simulink model "Solar_Panel"  (R2025b)
settings: Solver=VariableStepAuto  StartTime=0.0  StopTime=3600  RelTol=1e-3
undefined symbols (not defined in the file): J, Kd, Kf, Kg, Kt, L, R, sunPosition
libraries: slpidlib x1
settings Model: Creator=night  LastModifiedBy=night
settings DataIOCC: ExternalInput=[sunTime, sunPosition]  LoadExternalInput=on

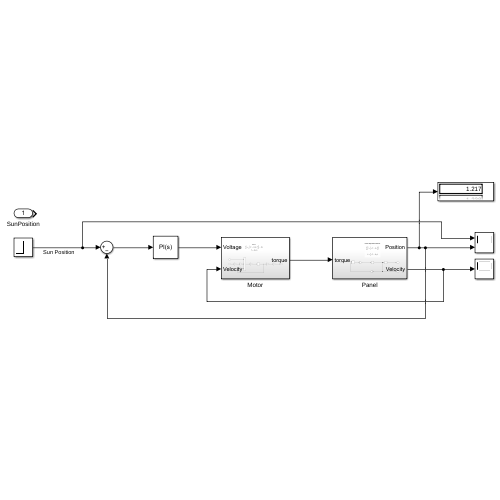
[thumbnail: Simulink's stored preview of the top-level diagram]
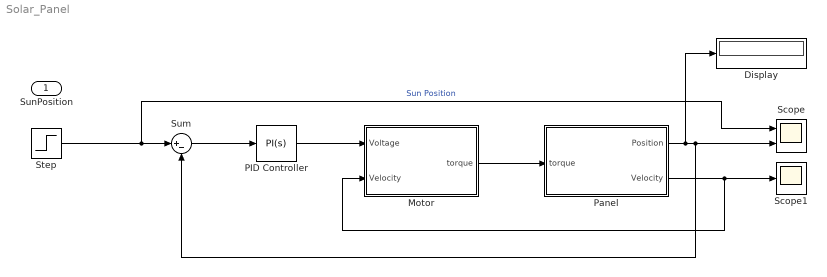
== system Solar_Panel ==
  SunPosition : Inport
  Display : Display
  Motor : Subsystem
  PID Controller : slpidlib/PID Controller  Controller=PI  Form=Parallel  TimeDomain=Continuous-time  UseExternalTs=off  SampleTime=-1  IntegratorMethod=Forward Euler  FilterMethod=Forward Euler  ControllerParametersSource=internal  P=240  I=180  UseKiTs=off  D=0  UseExternalDerivativeSource=off  N=100  UseFilter=on  TunerSelectOption=Transfer Function Based (PID Tuner App)  InitialConditionSource=internal  InitialConditionForIntegrator=0  InitialConditionForFilter=0  DifferentiatorICPrevScaledInput=0  ExternalReset=none  TrackingMode=off  Kt=1  LimitOutput=off  SatLimitsSource=internal  UpperSaturationLimit=inf  LowerSaturationLimit=-inf  LinearizeAsGain=on  AntiWindupMode=none  Kb=1  LimitIntegrator=off  UpperIntegratorSaturationLimit=inf  LowerIntegratorSaturationLimit=-inf  POutMin=[]  POutMax=[]  IOutMin=[]  IOutMax=[]  DOutMin=[]  DOutMax=[]  NOutMin=[]  NOutMax=[]  SumOutMin=[]  SumOutMax=[]  SaturationOutMin=[]  SaturationOutMax=[]  PParamMin=[]  PParamMax=[]  IParamMin=[]  IParamMax=[]  DParamMin=[]  DParamMax=[]  NParamMin=[]  NParamMax=[]  KbParamMin=[]  KbParamMax=[]  KtParamMin=[]  KtParamMax=[]  KbOutMin=[]  KbOutMax=[]  KtOutMin=[]  KtOutMax=[]  IntegratorOutMin=[]  IntegratorOutMax=[]  FilterOutMin=[]  FilterOutMax=[]  SumI1OutMin=[]  SumI1OutMax=[]  SumI2OutMin=[]  SumI2OutMax=[]  SumI3OutMin=[]  SumI3OutMax=[]  SumI4OutMin=[]  SumI4OutMax=[]  SumDOutMin=[]  SumDOutMax=[]  DifferentiatorOutMin=[]  DifferentiatorOutMax=[]  FilterDiffOutCoefMin=[]  FilterDiffOutCoefMax=[]  ReciprocalOutMin=[]  ReciprocalOutMax=[]  SumDenOutMin=[]  SumDenOutMax=[]  SumNumOutMin=[]  SumNumOutMax=[]  DivideOutMin=[]  DivideOutMax=[]  UdiffTsProdOutMin=[]  UdiffTsProdOutMax=[]  NTsProdOutMin=[]  NTsProdOutMax=[]  UintegralTsProdOutMin=[]  UintegralTsProdOutMax=[]  UngainTsProdOutMin=[]  UngainTsProdOutMax=[]  ClampingZeroOutDataTypeStr=Inherit: Inherit via back propagation  ClampingZeroOutMin=[]  ClampingZeroOutMax=[]  FilterDenConstantOutDataTypeStr=Inherit: Inherit via back propagation  FilterDenConstantOutMin=[]  FilterDenConstantOutMax=[]  PCopyOutDataTypeStr=Inherit: Inherit via back propagation  PCopyOutMin=[]  PCopyOutMax=[]  NCopyOutDataTypeStr=Inherit: Inherit via back propagation  NCopyOutMin=[]  NCopyOutMax=[]  IntegratorContinuousStateAttributes=''  IntegratorStateMustResolveToSignalObject=off  IntegratorRTWStateStorageClass=Auto  FilterContinuousStateAttributes=''  FilterStateMustResolveToSignalObject=off  FilterRTWStateStorageClass=Auto  ParallelPVariant=InternalParameters  IdealPVariant=Disabled  IVariant=InternalParameters  DVariant=Disabled  IntegratorVariant=Continuous  SatVariant=Disabled  AWVariant=Passthrough  PCopyVariant=Disabled  TRVariant=Disabled  FdbkBlocksVariant=Forward  IdealPFdbkVariant=Disabled  SatFdbkVariant=Disabled  DerivativeFilterVariant=Disabled  NVariant=Disabled  NCopyVariant=Disabled_SignalSpec  FilterICVariant=Disabled  IntegratorICVariant=InternalICs  ExternalResetVariant=Disabled  TRSumVariant=Passthrough  SumFdbkVariant=Disabled  SumVariant=Sum_PI  TsampFilterVariant=InternalTs  TsampNgainVariant=Passthrough  TsampIntegralVariant=Disabled_SignalSpec  ExternalSaturationOutDataTypeStr=Inherit: Same as second input  DerivativeSourceVariant=Disabled  PreIntVariant=InternalPreInt
  Panel : Subsystem
  Scope : Scope  NumInputPorts=2
      settings: Title=Solar Panel's Motor and Panel Assembly  ActiveDisplayYMinimum=-1  ActiveDisplayYMaximum=1
  Scope1 : Scope
      settings: ActiveDisplayYMinimum=-1  ActiveDisplayYMaximum=1
  Step : Step  After=sunPosition  SampleTime=0
  Sum : Sum  Inputs=|+-
  wires:
  Motor/1(torque) -> Panel/1(torque)
  Panel/1(Position) -> Display/1, Sum/2, Scope/2
  Panel/2(Velocity) -> Motor/2(Velocity), Scope1/1
  Step/1 -> Scope/1, Sum/1  "Sun Position"
  Sum/1 -> PID Controller/1
  PID Controller/1 -> Motor/1(Voltage)

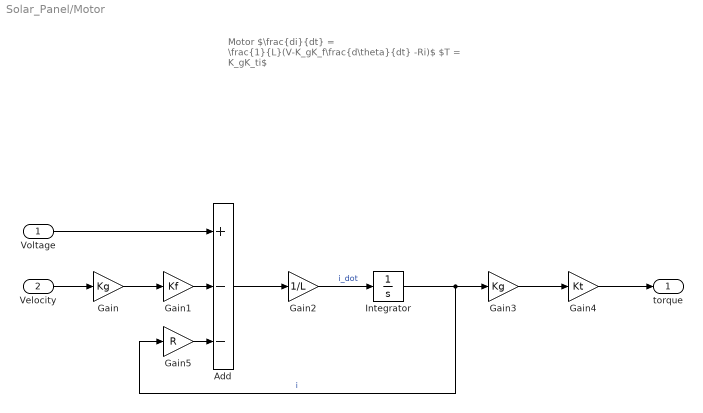
== system Solar_Panel/Motor ==
  note: Motor
      | $\frac{di}{dt} = \frac{1}{L}(V-K_gK_f\frac{d\theta}{dt} -Ri)$
      | $T = K_gK_ti$
  Voltage : Inport
  Velocity : Inport  Port=2
  Add : Sum  Inputs=+--
  Gain : Gain  Gain=Kg
  Gain1 : Gain  Gain=Kf
  Gain2 : Gain  Gain=1/L
  Gain3 : Gain  Gain=Kg
  Gain4 : Gain  Gain=Kt
  Gain5 : Gain  Gain=R
  Integrator : Integrator
  torque : Outport
  wires:
  Gain1/1 -> Add/2
  Velocity/1 -> Gain/1
  Add/1 -> Gain2/1
  Integrator/1 -> Gain5/1, Gain3/1  "i"
  Gain5/1 -> Add/3
  Gain3/1 -> Gain4/1
  Voltage/1 -> Add/1
  Gain/1 -> Gain1/1
  Gain2/1 -> Integrator/1  "i_dot"
  Gain4/1 -> torque/1

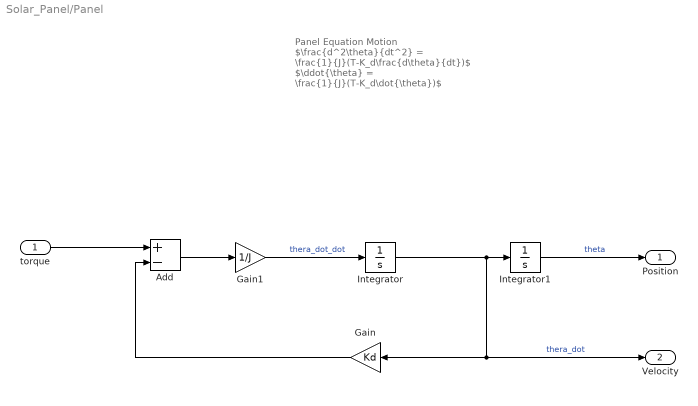
== system Solar_Panel/Panel ==
  note: Panel Equation Motion
      |
      | $\frac{d^2\theta}{dt^2} = \frac{1}{J}(T-K_d\frac{d\theta}{dt})$
      |
      | $\ddot{\theta} = \frac{1}{J}(T-K_d\dot{\theta})$
  torque : Inport
  Add : Sum  Inputs=+-
  Gain : Gain  Gain=Kd
  Gain1 : Gain  Gain=1/J
  Integrator : Integrator
  Integrator1 : Integrator
  Position : Outport
  Velocity : Outport  Port=2
  wires:
  Add/1 -> Gain1/1
  Gain1/1 -> Integrator/1  "thera_dot_dot"
  Integrator1/1 -> Position/1  "theta"
  Gain/1 -> Add/2
  torque/1 -> Add/1
  Integrator/1 -> Velocity/1, Gain/1, Integrator1/1  "thera_dot"
